simulink model "gm_lab2_floating_01slx"  (R2022a)
settings: Solver=VariableStepAuto  StartTime=0.0  StopTime=10.0  RelTol=1e-3
settings Model: Creator=Illia  LastModifiedBy=Illia
settings OptimizationCC: BlockReduction=off  ConditionallyExecuteInputs=off
settings DebuggingCC: InheritedTsInSrcMsg=none

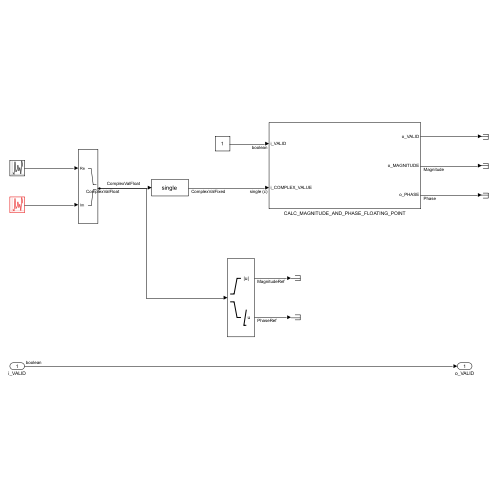
[thumbnail: Simulink's stored preview of the top-level diagram]
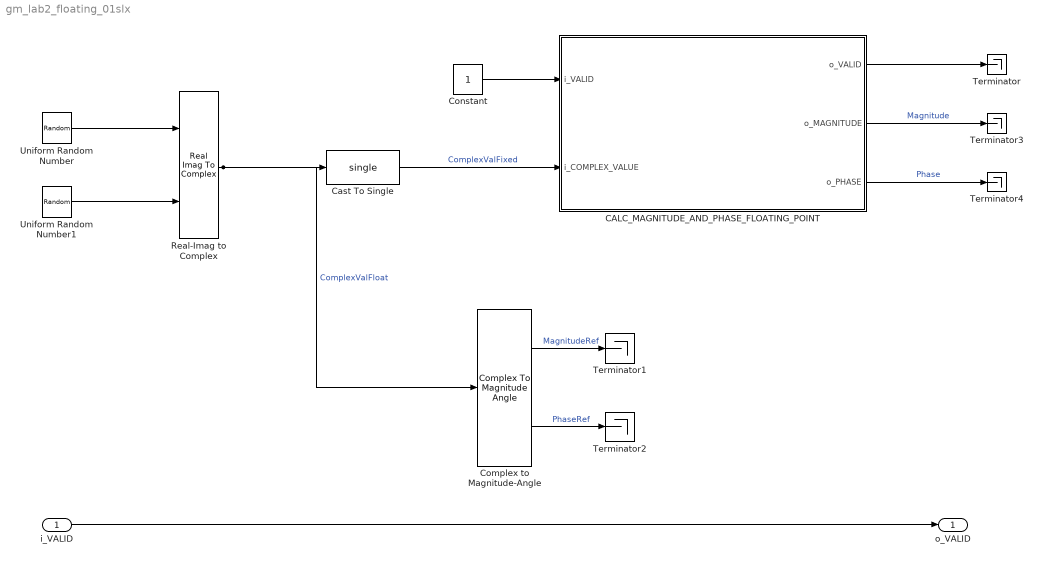
== system gm_lab2_floating_01slx ==
  i_VALID : Inport  OutDataTypeStr=boolean
  CALC_MAGNITUDE_AND_PHASE_FLOATING_POINT : Subsystem
  Cast To Single : DataTypeConversion  OutDataTypeStr=single  RndMeth=Nearest  SaturateOnIntegerOverflow=off
  Complex to Magnitude-Angle : ComplexToMagnitudeAngle
  Constant : Constant  OutDataTypeStr=boolean  SampleTime=1
  Real-Imag to Complex : RealImagToComplex
  Terminator{,1..4} (5 alike) : Terminator
  Uniform Random Number : UniformRandomNumber  Minimum=-4  Maximum=4  Seed=5  SampleTime=1
  Uniform Random Number1 : UniformRandomNumber  Seed=6  SampleTime=1
  o_VALID : Outport  VectorParamsAs1DForOutWhenUnconnected=off
  wires:
  CALC_MAGNITUDE_AND_PHASE_FLOATING_POINT/1(o_VALID) -> Terminator/1
  Uniform Random Number1/1 -> Real-Imag to Complex/2
  Complex to Magnitude-Angle/1 -> Terminator1/1  "MagnitudeRef"
  Uniform Random Number/1 -> Real-Imag to Complex/1
  Real-Imag to Complex/1 -> Complex to Magnitude-Angle/1, Cast To Single/1  "ComplexValFloat"
  CALC_MAGNITUDE_AND_PHASE_FLOATING_POINT/2(o_MAGNITUDE) -> Terminator3/1  "Magnitude"
  Complex to Magnitude-Angle/2 -> Terminator2/1  "PhaseRef"
  CALC_MAGNITUDE_AND_PHASE_FLOATING_POINT/3(o_PHASE) -> Terminator4/1  "Phase"
  Constant/1 -> CALC_MAGNITUDE_AND_PHASE_FLOATING_POINT/1(i_VALID)
  Cast To Single/1 -> CALC_MAGNITUDE_AND_PHASE_FLOATING_POINT/2(i_COMPLEX_VALUE)  "ComplexValFixed"
  i_VALID/1 -> o_VALID/1

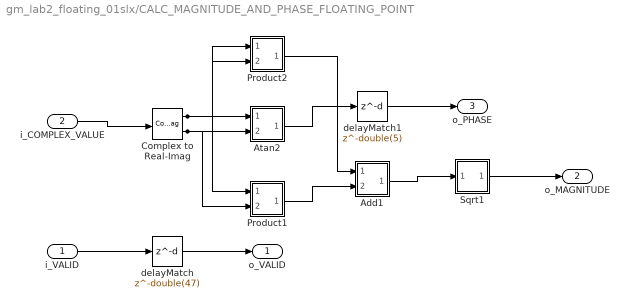
== system gm_lab2_floating_01slx/CALC_MAGNITUDE_AND_PHASE_FLOATING_POINT ==
  i_VALID : Inport  OutDataTypeStr=boolean  PortDimensions=1  SampleTime=1
  i_COMPLEX_VALUE : Inport  Port=2  OutDataTypeStr=single  PortDimensions=1  SampleTime=1
      settings: SignalType=complex
  Add1 : Subsystem
      mask Display: disp('NFP\nadd');
  Atan2 : Subsystem
      mask Display: disp('NFP\ntrig3');
  Complex to Real-Imag : ComplexToRealImag  SampleTime=1
  Product1 : Subsystem
      mask Display: disp('NFP\nmul');
  Product2 : Subsystem
      mask Display: disp('NFP\nmul');
  Sqrt1 : Subsystem
      mask Display: disp('NFP\nsqrt');
  delayMatch : Delay  DelayLength=double(47)  InitialCondition=0  SampleTime=1
  delayMatch1 : Delay  DelayLength=double(5)  InitialCondition=0  SampleTime=1
  o_VALID : Outport  SampleTime=1  VectorParamsAs1DForOutWhenUnconnected=off
  o_MAGNITUDE : Outport  Port=2  SampleTime=1
  o_PHASE : Outport  Port=3  SampleTime=1
  wires:
  delayMatch/1 -> o_VALID/1
  i_COMPLEX_VALUE/1 -> Complex to Real-Imag/1
  delayMatch1/1 -> o_PHASE/1
  Complex to Real-Imag/1 -> Product2/2(In2), Product2/1(In1), Atan2/2(In2)
  Complex to Real-Imag/2 -> Product1/2(In2), Product1/1(In1), Atan2/1(In1)
  Add1/1(Out1) -> Sqrt1/1(In1)
  Atan2/1(Out1) -> delayMatch1/1
  Product1/1(Out1) -> Add1/2(In2)
  Product2/1(Out1) -> Add1/1(In1)
  Sqrt1/1(Out1) -> o_MAGNITUDE/1
  i_VALID/1 -> delayMatch/1

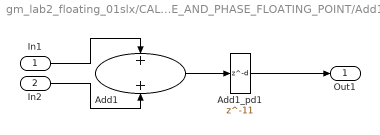
== system gm_lab2_floating_01slx/CALC_MAGNITUDE_AND_PHASE_FLOATING_POINT/Add1 ==
  In1 : Inport
  In2 : Inport  Port=2
  Add1 : Sum  OutDataTypeStr=single  SampleTime=1
  Add1_pd1 : Delay  DelayLength=11
  Out1 : Outport
  wires:
  In1/1 -> Add1/1
  In2/1 -> Add1/2
  Add1/1 -> Add1_pd1/1
  Add1_pd1/1 -> Out1/1

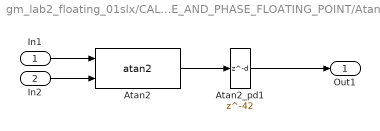
== system gm_lab2_floating_01slx/CALC_MAGNITUDE_AND_PHASE_FLOATING_POINT/Atan2 ==
  In1 : Inport
  In2 : Inport  Port=2
  Atan2 : Trigonometry  Operator=atan2  SampleTime=1
  Atan2_pd1 : Delay  DelayLength=42
  Out1 : Outport
  wires:
  In1/1 -> Atan2/1
  In2/1 -> Atan2/2
  Atan2/1 -> Atan2_pd1/1
  Atan2_pd1/1 -> Out1/1

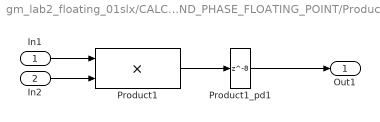
== system gm_lab2_floating_01slx/CALC_MAGNITUDE_AND_PHASE_FLOATING_POINT/Product1 ==
  In1 : Inport
  In2 : Inport  Port=2
  Product1 : Product  Inputs=**  OutDataTypeStr=single  SampleTime=1
  Product1_pd1 : Delay  DelayLength=8
  Out1 : Outport
  wires:
  In1/1 -> Product1/1
  In2/1 -> Product1/2
  Product1/1 -> Product1_pd1/1
  Product1_pd1/1 -> Out1/1

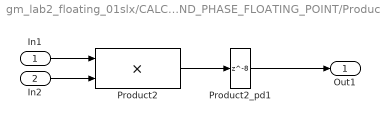
== system gm_lab2_floating_01slx/CALC_MAGNITUDE_AND_PHASE_FLOATING_POINT/Product2 ==
  In1 : Inport
  In2 : Inport  Port=2
  Product2 : Product  Inputs=**  OutDataTypeStr=single  SampleTime=1
  Product2_pd1 : Delay  DelayLength=8
  Out1 : Outport
  wires:
  In1/1 -> Product2/1
  In2/1 -> Product2/2
  Product2/1 -> Product2_pd1/1
  Product2_pd1/1 -> Out1/1

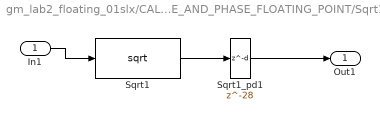
== system gm_lab2_floating_01slx/CALC_MAGNITUDE_AND_PHASE_FLOATING_POINT/Sqrt1 ==
  In1 : Inport
  Sqrt1 : Sqrt  SampleTime=1
  Sqrt1_pd1 : Delay  DelayLength=28
  Out1 : Outport
  wires:
  In1/1 -> Sqrt1/1
  Sqrt1/1 -> Sqrt1_pd1/1
  Sqrt1_pd1/1 -> Out1/1
